simulink model "sm_car"  (R2022a)
settings: Solver=ode23t  StartTime=0.0  StopTime=200  MaxStep=0.4  RelTol=1e-3  AbsTol=1e-3  EnableMultiTasking=on
PreLoadFcn:
  | disp('Loading default data for 2-axle vehicle and 1-axle trailer.')
  | if verLessThan('matlab', '9.11')
  |     load Vehicle_139
  |     Vehicle = Vehicle_139;
  |     load Trailer_01
  |     Trailer = Trailer_01;
  | else
  |     load Vehicle_189
  |     Vehicle = Vehicle_189;
  |     load Trailer_07
  |     Trailer = Trailer_07;
  | end
  | 
  | disp('Turning off MFEval warnings...')
  | disp('Solver:CoeffChecks:Eyk -- OFF')
  | disp('Solver:Limits:Exceeded -- OFF')
  | disp('Solver:CoeffChecks:Et -- OFF')
  | disp('Solver:CoeffChecks:Exa -- OFF')
  | 
  | warning('off','Solver:CoeffChecks:Eyk')
  | warning('off','Solver:Limits:Exceeded')
  | warning('off','Solver:CoeffChecks:Et')
  | warning('off','Solver:CoeffChecks:Exa')
  | %warning('off','Solver:Radius:NegativeRho')
  | 
  | % Due to usability issue in Repeating Sequence block
  | warning('off','Simulink:Masking:Invalid');
  | 
  | % Eliminate unnecessary warnings in inactive variants
  | % Warnings generated only if you click through inactive variant
  | warning('off','MATLAB:nonExistentField');
  | warning('off','Simulink:Parameters:BlkParamUndefined');
PostLoadFcn:
  | disp('Disabling trailer by default.')
  | set_param([bdroot '/Vehicle'],'popup_trailer','Off')
  | warning('off','sm:sli:setup:compile:LocalSolverNotSupported')
  | sm_car_config_maneuver(bdroot,'WOT Braking');
  | sm_car_config_vehicle(bdroot);
  | sm_car_config_logging(bdroot);
InitFcn:
  | sm_car_config_camera;
  | Vehicle = sm_car_vehcfg_checkConfig(Vehicle);
  | sm_car_check_tire_model(bdroot);
  | addpath('C:\MasterThesis_CEVT\code\casadi-windows-matlabR2016a-v3.5.5')
  | addpath('C:\MasterThesis_CEVT\code')
  | addpath('C:\MasterThesis_CEVT\code\python scripts')
StartFcn:
  | tic;
StopFcn:
  | Elapsed_Sim_Time = toc;
  | % disp(['Elapsed Sim Time = ' num2str(Elapsed_Sim_Time)]);
  | % Run script that exports relevant simulation data to json
  | simToJson
undefined symbols (not defined in the file or in its folder): Control, Driver, Maneuver
libraries: sm_car_lib x22, simulink x17, sm_lib x3, Vehicle_Visualization x3, Driver_Long_Lat_Stanley x2, Maneuver_Get_Pose x2, Camera_Frame_Definitions x1, Control_FuelCell1Motor x1, slpidlib x1, Driver_Drive_Cycle x1, Driver_Gamepad_Xbox x1, Driver_Open_Loop x1
(part 2 of 3)

== system sm_car/Road/Input fWindTrailer ==
  Bus Creator1 : BusCreator  Inputs=3
  Demux : Demux  Outputs=3
  Scope : Scope
  Step : Step  Time=dWind  After=fWind  SampleTime=0
  Step1 : Step  Time=dWind+tWind  After=fWind  SampleTime=0
  Sum : Sum  Inputs=|+-
  fWind : Outport  VectorParamsAs1DForOutWhenUnconnected=off
  wires:
  Bus Creator1/1 -> fWind/1
  Demux/3 -> Bus Creator1/3  "fz"
  Demux/1 -> Bus Creator1/1  "fx"
  Demux/2 -> Bus Creator1/2  "fy"
  Sum/1 -> Scope/1, Demux/1  "fxyz"
  Step1/1 -> Sum/2
  Step/1 -> Sum/1

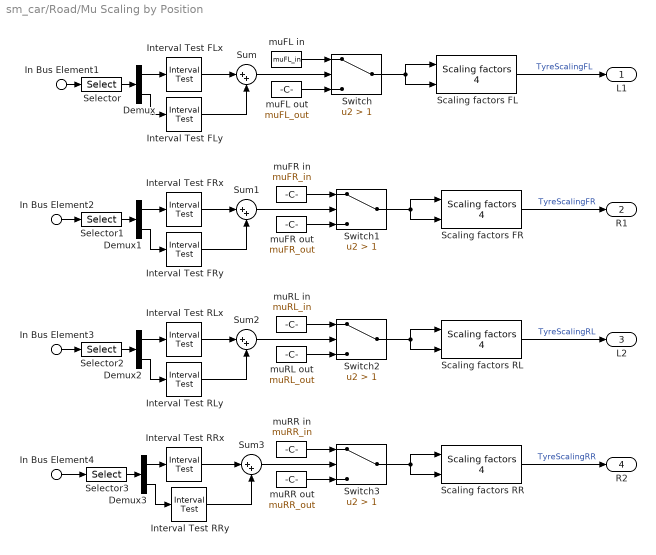
== system sm_car/Road/Mu Scaling by Position ==
  In Bus Element1 : Inport  PortName=Chassis  Element=WhlL1.xyz
  In Bus Element2 : Inport  PortName=Chassis  Element=WhlR1.xyz
  In Bus Element3 : Inport  PortName=Chassis  Element=WhlL2.xyz
  In Bus Element4 : Inport  PortName=Chassis  Element=WhlR2.xyz
  Demux{,1..3} (4 alike) : Demux  Outputs=2
  Interval Test FLx : simulink/Logic and Bit Operations/Interval Test  IntervalClosedRight=on  uplimit=intvX_FL_end  IntervalClosedLeft=on  lowlimit=intvX_FL_start  OutDataTypeStr=uint8
  Interval Test FLy : simulink/Logic and Bit Operations/Interval Test  IntervalClosedRight=on  uplimit=intvY_FL_end  IntervalClosedLeft=on  lowlimit=intvY_FL_start  OutDataTypeStr=uint8
  Interval Test FRx : simulink/Logic and Bit Operations/Interval Test  IntervalClosedRight=on  uplimit=intvX_FR_end  IntervalClosedLeft=on  lowlimit=intvX_FR_start  OutDataTypeStr=uint8
  Interval Test FRy : simulink/Logic and Bit Operations/Interval Test  IntervalClosedRight=on  uplimit=intvY_FR_end  IntervalClosedLeft=on  lowlimit=intvY_FR_start  OutDataTypeStr=uint8
  Interval Test RLx : simulink/Logic and Bit Operations/Interval Test  IntervalClosedRight=on  uplimit=intvX_RL_end  IntervalClosedLeft=on  lowlimit=intvX_RL_start  OutDataTypeStr=uint8
  Interval Test RLy : simulink/Logic and Bit Operations/Interval Test  IntervalClosedRight=on  uplimit=intvY_RL_end  IntervalClosedLeft=on  lowlimit=intvY_RL_start  OutDataTypeStr=uint8
  Interval Test RRx : simulink/Logic and Bit Operations/Interval Test  IntervalClosedRight=on  uplimit=intvX_RR_end  IntervalClosedLeft=on  lowlimit=intvX_RR_start  OutDataTypeStr=uint8
  Interval Test RRy : simulink/Logic and Bit Operations/Interval Test  IntervalClosedRight=on  uplimit=intvY_RR_end  IntervalClosedLeft=on  lowlimit=intvY_RR_start  OutDataTypeStr=uint8
  Scaling factors FL : sm_car_lib/Tires/Scaling factors 4  LKX=1  LKY=1  LKYC=1  LTR=1  LKZC=1
  Scaling factors FR : sm_car_lib/Tires/Scaling factors 4  LKX=1  LKY=1  LKYC=1  LTR=1  LKZC=1
  Scaling factors RL : sm_car_lib/Tires/Scaling factors 4  LKX=1  LKY=1  LKYC=1  LTR=1  LKZC=1
  Scaling factors RR : sm_car_lib/Tires/Scaling factors 4  LKX=1  LKY=1  LKYC=1  LTR=1  LKZC=1
  Selector{,1..3} (4 alike) : Selector  InputPortWidth=3  IndexOptions=Index vector (dialog)  Indices=[1 2]  OutputSizes=1
  Sum{,1..3} (4 alike) : Sum  Inputs=|++
  Switch : Switch  Criteria=u2 > Threshold  Threshold=1  ZeroCross=off  SaturateOnIntegerOverflow=off  InputSameDT=off
  Switch1 : Switch  Criteria=u2 > Threshold  Threshold=1  SaturateOnIntegerOverflow=off  InputSameDT=off
  Switch2 : Switch  Criteria=u2 > Threshold  Threshold=1  SaturateOnIntegerOverflow=off  InputSameDT=off
  Switch3 : Switch  Criteria=u2 > Threshold  Threshold=1  SaturateOnIntegerOverflow=off  InputSameDT=off
  muFL in : Constant  Value=muFL_in
  muFL out : Constant  Value=muFL_out
  muFR in : Constant  Value=muFR_in
  muFR out : Constant  Value=muFR_out
  muRL in : Constant  Value=muRL_in
  muRL out : Constant  Value=muRL_out
  muRR in : Constant  Value=muRR_in
  muRR out : Constant  Value=muRR_out
  L1 : Outport  VectorParamsAs1DForOutWhenUnconnected=off
  R1 : Outport  Port=2  VectorParamsAs1DForOutWhenUnconnected=off
  L2 : Outport  Port=3  VectorParamsAs1DForOutWhenUnconnected=off
  R2 : Outport  Port=4  VectorParamsAs1DForOutWhenUnconnected=off
  wires:
  Demux/1 -> Interval Test FLx/1
  Interval Test RRx/1 -> Sum3/1
  Demux3/2 -> Interval Test RRy/1
  Demux3/1 -> Interval Test RRx/1
  Sum3/1 -> Switch3/2
  Selector3/1 -> Demux3/1
  In Bus Element4/1 -> Selector3/1
  Interval Test RRy/1 -> Sum3/2
  Demux2/2 -> Interval Test RLy/1
  Selector2/1 -> Demux2/1
  Demux2/1 -> Interval Test RLx/1
  Interval Test RLy/1 -> Sum2/2
  Sum2/1 -> Switch2/2
  In Bus Element3/1 -> Selector2/1
  Interval Test RLx/1 -> Sum2/1
  Interval Test FRy/1 -> Sum1/2
  Selector1/1 -> Demux1/1
  Demux1/2 -> Interval Test FRy/1
  Sum1/1 -> Switch1/2
  Demux1/1 -> Interval Test FRx/1
  Interval Test FRx/1 -> Sum1/1
  Interval Test FLx/1 -> Sum/1
  Interval Test FLy/1 -> Sum/2
  Sum/1 -> Switch/2
  Demux/2 -> Interval Test FLy/1
  Selector/1 -> Demux/1
  muRR out/1 -> Switch3/3
  muRR in/1 -> Switch3/1
  Switch3/1 -> Scaling factors RR/2, Scaling factors RR/1
  Scaling factors RR/1 -> R2/1  "TyreScalingRR"
  Scaling factors RL/1 -> L2/1  "TyreScalingRL"
  Switch2/1 -> Scaling factors RL/1, Scaling factors RL/2
  muRL in/1 -> Switch2/1
  muRL out/1 -> Switch2/3
  muFR out/1 -> Switch1/3
  In Bus Element2/1 -> Selector1/1
  muFR in/1 -> Switch1/1
  Switch1/1 -> Scaling factors FR/2, Scaling factors FR/1
  Scaling factors FR/1 -> R1/1  "TyreScalingFR"
  Scaling factors FL/1 -> L1/1  "TyreScalingFL"
  Switch/1 -> Scaling factors FL/1, Scaling factors FL/2
  muFL out/1 -> Switch/3
  muFL in/1 -> Switch/1
  In Bus Element1/1 -> Selector/1

== system sm_car/Scopes/Subsystem ==
  In1 : Inport
  Bus Selector4 : BusSelector  OutputSignals=Chassis.Body.CG.vx,Chassis.Body.CG.vy,World.vx,World.vy,World.x,World.y
  Mux : Mux  Inputs=2
  Mux1 : Mux  Inputs=2
  Mux2 : Mux  Inputs=2
  Vel in xy plane : Fcn  Expr=sqrt(u(1)^2+u(2)^2)
  Vel in xy plane1 : Fcn  Expr=sqrt(u(1)^2+u(2)^2)
  Vel in xy plane2 : Fcn  Expr=sqrt(u(1)^2+u(2)^2)
  vBody : Outport  VectorParamsAs1DForOutWhenUnconnected=off
  vWorld : Outport  Port=2  VectorParamsAs1DForOutWhenUnconnected=off
  xWorld : Outport  Port=3  VectorParamsAs1DForOutWhenUnconnected=off
  wires:
  Bus Selector4/3 -> Mux1/1  "<vx>"
  Bus Selector4/4 -> Mux1/2  "<vy>"
  Bus Selector4/1 -> Mux/1  "<vx>"
  Vel in xy plane1/1 -> vWorld/1  "speed"
  In1/1 -> Bus Selector4/1
  Mux1/1 -> Vel in xy plane1/1
  Mux/1 -> Vel in xy plane/1
  Vel in xy plane/1 -> vBody/1  "speed"
  Bus Selector4/2 -> Mux/2  "<vy>"
  Mux2/1 -> Vel in xy plane2/1
  Bus Selector4/6 -> Mux2/2  "<y>"
  Bus Selector4/5 -> Mux2/1  "<x>"
  Vel in xy plane2/1 -> xWorld/1  "speed"

== system sm_car/Vehicle/Vehicle Constraint ==
  No Constraint : Subsystem  VariantControl=NoConstraint
  No Yaw : Subsystem  VariantControl=NoYaw
  F : PMIOPort  Side=Right
  B : PMIOPort  Port=2  Side=Left

== system sm_car/Visualization/Dashboard ==
  VehBus : Inport
  DrvBus : Inport  Port=2
  Accelerator Pedal : LinearGaugeBlock  LabelPosition=Hide  ScaleMax=1
  Brake Pedal : LinearGaugeBlock  ScaleMax=1
  Bus Selector : BusSelector  OutputSignals=Chassis.Body.CG.vx
  Bus Selector2 : BusSelector  OutputSignals=aSteerWheel,rAccelPedal,rBrakePedal
  Gain : Gain  Gain=180/pi
  Gain1 : Gain  Gain=3.6
  Speed (kph) : CustomWebBlock  LabelPosition=Hide  ShowInitialText=on  Configuration="{\"components\":[{\"name\":\"CircularScaleComponent\",\"settings\":{\"bounds\":{\"max\":150,\"min\":0,\"tickInterval\":\"auto\"},\"direction\":\"cw\",\"flipLimits\":0,\"innerRadius\":0.46396628518311167,\"internalTickHeightScaleFactor\":1,\"labelColor\":[250,245,200],\"labelFont\":{\"font\":\"Arial\",\"fontSize\":12},\"labelRadius\":0.36,\"labelTransparency\":1,\"minorTickHeightScaleFactor\":0.2,\"needleImage\":{\"size\":[1890,567],\"src\":\"data:image\\/svg+xml;base64,PD94bWwgdmVyc2lvbj0iMS4wIiBlbmNvZGluZz0iVVRGLTgiIHN0YW5kYWxvbmU9Im5vIj8+CjxzdmcKICAgeG1sbnM6ZGM9Imh0dHA6Ly9wdXJsLm9yZy9kYy9lbGVtZW50cy8xLjEvIgogICB4bWxuczpjYz0iaHR0cDovL2NyZWF0aXZlY29tbW9ucy5vcmcvbnMjIgogICB4bWxuczpyZGY9Imh0dHA6Ly93d3cudzMub3JnLzE5OTkvMDIvMjItcmRmLXN5bnRheC1ucyMiCiAgIHhtbG5zOnN2Zz0iaHR0cDovL3d3dy53My5vcmcvMjAwMC9zdmciCiAgIHhtbG5zPSJodHRwOi8vd3d3LnczLm9yZy8yMDAwL3N2ZyIKICAgeG1sbnM6 ...(+4096 chars)\"},\"needleOffset\":[0.14,0],\"needleOrientation\":-45,\"needleRotation\":180,\"needleSize\":{\"height\":0.13,\"width\":0.41},\"outerRadius\":0.6228849068763098,\"position\":[0,0,1,1],\"scaleAngle\":299.999999999988,\"scaleAngleOffset\":119.46147497096791,\"scaleColors\":[],\"scaleColorsSize\":0.2,\"scalePosition\":[0,0,1,1],\"showLabels\":1,\"showMinorTicks\":1,\"showSpanLine\":1,\"showTicks\":1,\"tickColor\":[250,245,200],\"tickTransparency\":1,\"valueBarColor\":[23,89,176],\"valueBarPosition\":[0,0,1,1],\"valueBarSize\":0.2,\"valueBarTransparency\":1}},{\"name\":\"BackgroundImageComponent\",\"settings\":{\"image\":{\"size\":[500,500],\"src\":\"data:image\\/svg+xml;base64,PD94bWwgdmVyc2lvbj0iMS4wIiBlbmNvZGluZz0iVVRGLTgiIHN0YW5kYWxvbmU9Im5vIj8+CjwhLS0gR2VuZXJhdG9yOiBBZG9iZSBJbGx1c3RyYXRvciAxOS4yLjEsIFNWRyBFeHBvcnQgUGx1Zy1JbiAuIFNWRyBWZXJzaW9uOiA2LjAwIEJ1aWxkIDApICAtLT4KCjxzdmcKICAgeG1sbnM6ZGM9Imh0dHA6Ly9wdXJsLm9yZy9kYy9lbGVtZW50cy8xLjEvIgogICB4bWxuczpjYz0iaHR0cDovL2NyZWF0aXZlY29tbW9ucy5vcmcvbnMjIgogICB4bWxuczpyZGY9Imh0dHA6Ly93d3cudzMub3JnLzE5OTkvMDIvMjItcmRmLXN5bnRh ...(+9660 chars)\",\"srcOrientation\":\"horizontal\"},\"position\":[0,0,1,1],\"scaleMode\":\"0\"}},{\"name\":\"ForegroundImageComponent\",\"settings\":{\"image\":{\"size\":[0,0],\"src\":\"default\",\"srcOrientation\":[]},\"isForeground\":1,\"position\":[0,0,1,1],\"scaleMode\":\"0\"}}],\"settings\":{\"BindingType\":\"signal\",\"backgroundOffset\":0.14,\"backgroundOpacity\":1,\"fixedAspectRatio\":\"on\",\"orientation\":\"horizontal\",\"showBackgroundColor\":0},\"type\":\"CircularGauge\"}"
  Steering Wheel Angle : SemiCircularGaugeBlock  LabelPosition=Hide  ScaleMin=-80  ScaleMax=80  TickInterval=20
  Terminator{,1..3} (4 alike) : Terminator
  wires:
  VehBus/1 -> Bus Selector/1
  DrvBus/1 -> Bus Selector2/1
  Bus Selector/1 -> Gain1/1  "<vx>"
  Gain/1 -> Terminator1/1  "aSteerWheel deg"
  Bus Selector2/3 -> Terminator3/1  "<rBrakePedal>"
  Bus Selector2/1 -> Gain/1  "<aSteerWheel>"
  Bus Selector2/2 -> Terminator2/1  "<rAccelPedal>"
  Gain1/1 -> Terminator/1  "Speed (kph)"

== system sm_car/Visualization/Unreal ==
  "xyz " : Inport
  "rpy " : Inport  Port=2
  "ws " : Inport  Port=3
  "aCamber " : Inport  Port=4
  "aSteerWheel " : Inport  Port=5
  Animation Off : Subsystem  VariantControl=Off
  Animation On : Subsystem  VariantControl=On

== system sm_car/Visualization/XY Plot ==
  "VehBus " : Inport
  "DrvBus " : Inport  Port=2
  XY Plot Off : Subsystem  VariantControl=Off
  XY Plot On : Vehicle_Visualization/XY Plot  SystemSampleTime=-1  VariantControl=On  VariantActivationTime=update diagram  Latency=0  AutoFrameSizeCalculation=off

== system sm_car/Controller/Battery 2 Motor/Accel Torque Request ==
  note: Convert Accelerator Pedal Position to Torque Command
      | using Motor Torque Speed Curve
  MotSpdA1 : Inport
  MotSpdA2 : Inport  Port=2
  AccelPdl : Inport  Port=3
  MaxMotTrqVsSpdA1 : Lookup_n-D  NumberOfTableDimensions=1  BreakpointsForDimension1=Control.MotorA1.TorqueSpd.w.Value %Mot.w_eff_bp_EV_rear  Table=Control.MotorA1.TorqueSpd.trq.Value % Mot.T_t_EV_rear  ExtrapMethod=Clip  UseLastTableValue=on  InternalRulePriority=Speed  OutDataTypeStr=Inherit: Inherit from 'Table data'  RndMeth=Simplest
  MaxMotTrqVsSpdA2 : Lookup_n-D  NumberOfTableDimensions=1  BreakpointsForDimension1=Control.MotorA2.TorqueSpd.w.Value  Table=Control.MotorA2.TorqueSpd.trq.Value  ExtrapMethod=Clip  UseLastTableValue=on  InternalRulePriority=Speed  OutDataTypeStr=Inherit: Inherit from 'Table data'  RndMeth=Simplest
  Mux : Mux  Inputs=2
  Product1 : Product
  Product2 : Product
  rads_to_rpm : Gain  Gain=30/pi
  rads_to_rpm1 : Gain  Gain=30/pi
  TrqCmd : Outport  VectorParamsAs1DForOutWhenUnconnected=off
  wires:
  rads_to_rpm/1 -> MaxMotTrqVsSpdA1/1
  MotSpdA1/1 -> rads_to_rpm/1
  AccelPdl/1 -> Product1/1, Product2/1
  MaxMotTrqVsSpdA1/1 -> Product1/2
  Product1/1 -> Mux/1
  MotSpdA2/1 -> rads_to_rpm1/1
  rads_to_rpm1/1 -> MaxMotTrqVsSpdA2/1
  MaxMotTrqVsSpdA2/1 -> Product2/2
  Product2/1 -> Mux/2
  Mux/1 -> TrqCmd/1

== system sm_car/Controller/Battery 2 Motor/Accel//Decel ==
  TrqCmdDec : Inport
  TrqCmdAcc : Inport  Port=2
  AccelPdl : Inport  Port=3
  Accel Decel Switch : Switch  Criteria=u2 > Threshold  SaturateOnIntegerOverflow=off  InputSameDT=off
  Compare To Constant : simulink/Logic and Bit Operations/Compare To Constant  relop=>  const=1e-2  OutDataTypeStr=boolean  ZeroCross=off
  Demux : Demux  Outputs=2
  MotTrqA1 : Outport  VectorParamsAs1DForOutWhenUnconnected=off
  MotTrqA2 : Outport  Port=2  VectorParamsAs1DForOutWhenUnconnected=off
  wires:
  TrqCmdDec/1 -> Accel Decel Switch/3
  Accel Decel Switch/1 -> Demux/1
  TrqCmdAcc/1 -> Accel Decel Switch/1
  AccelPdl/1 -> Compare To Constant/1
  Compare To Constant/1 -> Accel Decel Switch/2
  Demux/1 -> MotTrqA1/1
  Demux/2 -> MotTrqA2/1

== system sm_car/Controller/Battery 2 Motor/Battery Management System ==
  note: Behaviorial BMS System. Limits battery charge / discharge power based on SOC.
      |
      | Charge/Discharge Limits and curves can be adjusted if using a larger battery pack
      | or motor power is changed.
  SOC : Inport
  ChrgLmt : Lookup_n-D  NumberOfTableDimensions=1  BreakpointsForDimension1=Control.Battery.SOC_bpt  Table=Control.Battery.ChrgLmt_bpt  ExtrapMethod=Clip  UseLastTableValue=on  InternalRulePriority=Speed  RndMeth=Simplest
  DischrgLmt : Lookup_n-D  NumberOfTableDimensions=1  BreakpointsForDimension1=Control.Battery.SOC_bpt  Table=Control.Battery.DischrgLmt_bpt  ExtrapMethod=Clip  UseLastTableValue=on  InternalRulePriority=Speed  RndMeth=Simplest
  MaxChrg : Constant  Value=Control.Battery.BattChrgMax
  MaxDischrg : Constant  Value=Control.Battery.BattDischrgMax
  Product : Product
  Product1 : Product
  PwrLimtDis : Outport  VectorParamsAs1DForOutWhenUnconnected=off
  PwrLimitChg : Outport  Port=2  VectorParamsAs1DForOutWhenUnconnected=off
  wires:
  DischrgLmt/1 -> Product/1
  ChrgLmt/1 -> Product1/1
  Product1/1 -> PwrLimitChg/1
  Product/1 -> PwrLimtDis/1
  MaxDischrg/1 -> Product/2
  MaxChrg/1 -> Product1/2
  SOC/1 -> ChrgLmt/1, DischrgLmt/1

== system sm_car/Controller/Battery 2 Motor/Brake Pressure Request ==
  note: Converts Brake Pedal Position to Deceleration Request
  DecelPdl : Inport
  Park : Inport  Port=2
  Constant1 : Constant
  Switch : Switch  Criteria=u2 > Threshold  ZeroCross=off  SaturateOnIntegerOverflow=off  InputSameDT=off
  BrkDecelReq : Outport  VectorParamsAs1DForOutWhenUnconnected=off
  wires:
  Park/1 -> Switch/2
  Switch/1 -> BrkDecelReq/1
  Constant1/1 -> Switch/1
  DecelPdl/1 -> Switch/3

== system sm_car/Controller/Battery 2 Motor/Per wheel ==
  pBrake : Inport
  Bus Creator4 : BusCreator  Inputs=4
  Gain1 : Gain  Gain=0.6
  Gain2 : Gain  Gain=0.6
  Gain3 : Gain  Gain=0.4
  Gain4 : Gain  Gain=0.4
  Gain5 : Gain  Gain=0.5
  Transfer Fcn : TransferFcn  Denominator=[0.01 1]
  p : Outport  VectorParamsAs1DForOutWhenUnconnected=off
  wires:
  Gain4/1 -> Bus Creator4/4  "pBrakeR2"
  Gain3/1 -> Bus Creator4/3  "pBrakeL2"
  Gain1/1 -> Bus Creator4/2  "pBrakeR1"
  Bus Creator4/1 -> p/1
  pBrake/1 -> Transfer Fcn/1
  Gain2/1 -> Bus Creator4/1  "pBrakeL1"
  Gain5/1 -> Gain2/1, Gain1/1, Gain3/1, Gain4/1  "pBrakeL1"
  Transfer Fcn/1 -> Gain5/1

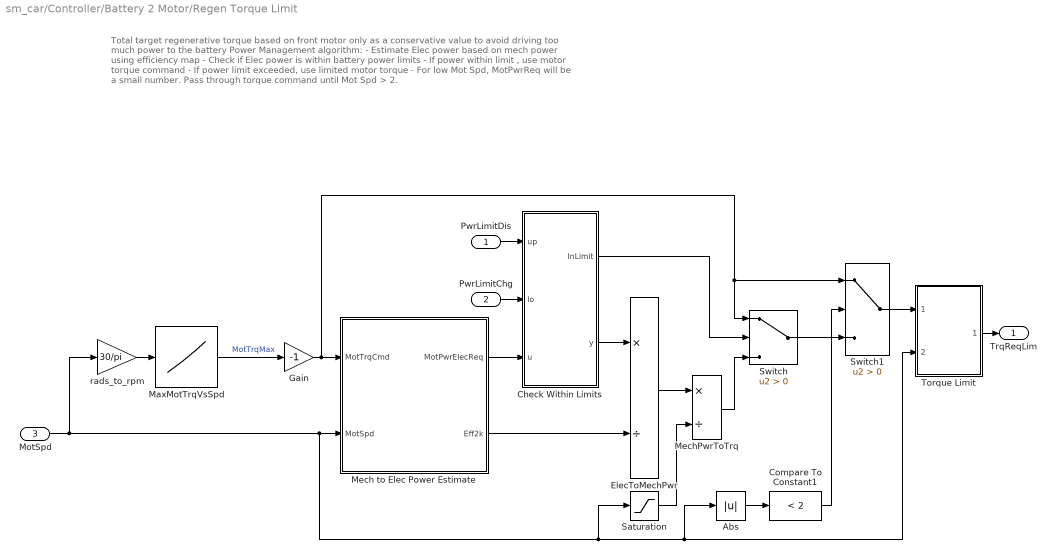
== system sm_car/Controller/Battery 2 Motor/Regen Torque Limit ==
  note: Total target regenerative torque based on front motor only as a conservative value to avoid driving too much power to the battery
      |
      | Power Management algorithm:
      | - Estimate Elec power based on mech power using efficiency map
      | - Check if Elec power is within battery power limits
      | - If power within limit , use motor torque command
      | - If power limit exceeded, use limited motor torque
      | - For low Mot Spd, MotPwrReq will be a small number.  Pass through torque command until Mot Spd > 2.
  PwrLimitDis : Inport
  "PwrLimitChg " : Inport  Port=2
  MotSpd : Inport  Port=3
  Abs : Abs  ZeroCross=off  SaturateOnIntegerOverflow=off
  Check Within Limits : Subsystem
  Compare To Constant1 : simulink/Logic and Bit Operations/Compare To Constant  relop=<  const=2  OutDataTypeStr=boolean  ZeroCross=off
  ElecToMechPwr : Product  Inputs=*/
  Gain : Gain  Gain=-1
  MaxMotTrqVsSpd : Lookup_n-D  NumberOfTableDimensions=1  BreakpointsForDimension1=Control.MotorA1.TorqueSpd.w.Value  Table=Control.MotorA1.TorqueSpd.trq.Value  ExtrapMethod=Clip  UseLastTableValue=on  InternalRulePriority=Speed  OutDataTypeStr=Inherit: Inherit from 'Table data'  RndMeth=Simplest
  Mech to Elec Power Estimate : Subsystem
  MechPwrToTrq : Product  Inputs=*/
  Saturation : Saturate  UpperLimit=inf  LowerLimit=2
  Switch : Switch  Criteria=u2 > Threshold  ZeroCross=off  SaturateOnIntegerOverflow=off  InputSameDT=off
  Switch1 : Switch  Criteria=u2 > Threshold  ZeroCross=off  SaturateOnIntegerOverflow=off  InputSameDT=off
  Torque Limit : Subsystem
  rads_to_rpm : Gain  Gain=30/pi
  "TrqReqLim " : Outport  VectorParamsAs1DForOutWhenUnconnected=off
  wires:
  Switch1/1 -> Torque Limit/1(MotTrq)
  Torque Limit/1(MotReqCmd) -> "TrqReqLim "/1
  Mech to Elec Power Estimate/2(Eff2k) -> ElecToMechPwr/2
  PwrLimitDis/1 -> Check Within Limits/1(up)
  "PwrLimitChg "/1 -> Check Within Limits/2(lo)
  Gain/1 -> Mech to Elec Power Estimate/1(MotTrqCmd), Switch/1, Switch1/1
  Check Within Limits/1(InLimit) -> Switch/2
  Check Within Limits/2(y) -> ElecToMechPwr/1
  Mech to Elec Power Estimate/1(MotPwrElecReq) -> Check Within Limits/3(u)
  Switch/1 -> Switch1/3
  Abs/1 -> Compare To Constant1/1
  Compare To Constant1/1 -> Switch1/2
  Saturation/1 -> MechPwrToTrq/2
  MechPwrToTrq/1 -> Switch/3
  ElecToMechPwr/1 -> MechPwrToTrq/1
  rads_to_rpm/1 -> MaxMotTrqVsSpd/1
  MaxMotTrqVsSpd/1 -> Gain/1  "MotTrqMax"
  MotSpd/1 -> Torque Limit/2(MotSpd), Abs/1, Saturation/1, Mech to Elec Power Estimate/2(MotSpd), rads_to_rpm/1

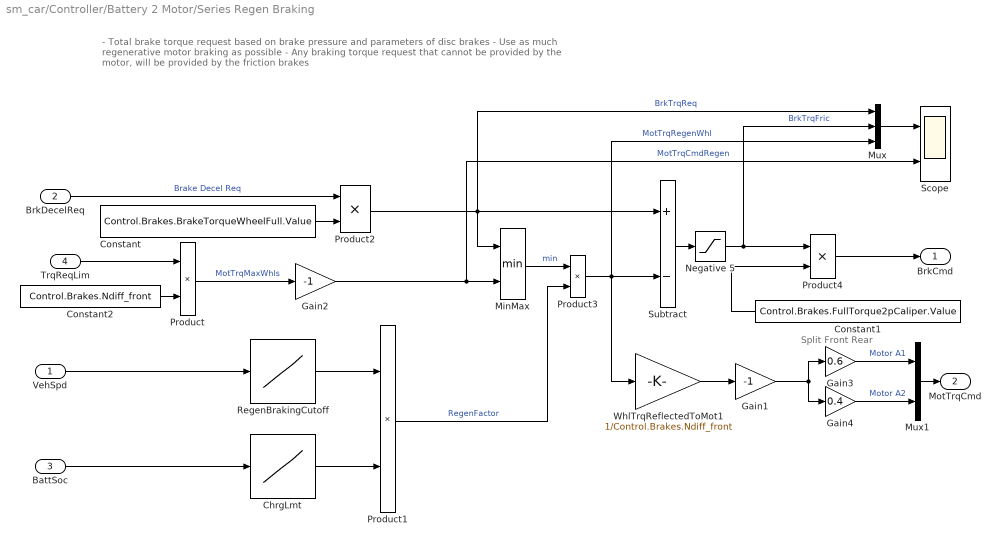
== system sm_car/Controller/Battery 2 Motor/Series Regen Braking ==
  note: Split Front Rear
  note: - Total brake torque request based on brake pressure and parameters of disc brakes
      | - Use as much regenerative motor braking as possible
      | - Any braking torque request that cannot be provided by the motor, will be provided by the friction brakes
  VehSpd : Inport
  BrkDecelReq : Inport  Port=2
  BattSoc : Inport  Port=3
  TrqReqLim : Inport  Port=4
  ChrgLmt : Lookup_n-D  NumberOfTableDimensions=1  BreakpointsForDimension1=Control.Battery.SOC_bpt  Table=Control.Battery.ChrgLmt_bpt  ExtrapMethod=Clip  UseLastTableValue=on  InternalRulePriority=Speed  RndMeth=Simplest
  Constant : Constant  Value=Control.Brakes.BrakeTorqueWheelFull.Value
  Constant1 : Constant  Value=Control.Brakes.FullTorque2pCaliper.Value
  Constant2 : Constant  Value=Control.Brakes.Ndiff_front
  Gain1 : Gain  Gain=-1
  Gain2 : Gain  Gain=-1
  Gain3 : Gain  Gain=0.6
  Gain4 : Gain  Gain=0.4
  MinMax : MinMax  Inputs=2
  Mux : Mux  Inputs=3
  Mux1 : Mux  Inputs=2
  Negative 5 : Saturate  UpperLimit=inf  LowerLimit=0  ZeroCross=off
  Product{,1..3} (4 alike) : Product
  Product4 : Product  Inputs=**
  RegenBrakingCutoff : Lookup_n-D  NumberOfTableDimensions=1  BreakpointsForDimension1=Control.Power.RegenBrkSpd_bpt  Table=Control.Power.RegenBrkCutOff  ExtrapMethod=Clip  UseLastTableValue=on  InternalRulePriority=Speed  RndMeth=Simplest
  Scope : Scope  NumInputPorts=2
  Subtract : Sum  Inputs=+-
  WhlTrqReflectedToMot1 : Gain  Gain=1/Control.Brakes.Ndiff_front
  " BrkCmd" : Outport  VectorParamsAs1DForOutWhenUnconnected=off
  " MotTrqCmd" : Outport  Port=2  VectorParamsAs1DForOutWhenUnconnected=off
  wires:
  Product4/1 -> " BrkCmd"/1
  Negative 5/1 -> Product4/1, Mux/2  "BrkTrqFric"
  BattSoc/1 -> ChrgLmt/1
  Subtract/1 -> Negative 5/1
  Product1/1 -> Product3/2  "RegenFactor"
  RegenBrakingCutoff/1 -> Product1/1
  VehSpd/1 -> RegenBrakingCutoff/1
  ChrgLmt/1 -> Product1/2
  MinMax/1 -> Product3/1  "min"
  Product2/1 -> MinMax/1, Subtract/1, Mux/1  "BrkTrqReq"
  BrkDecelReq/1 -> Product2/1  "Brake Decel Req"
  Constant/1 -> Product2/2
  Constant1/1 -> Product4/2
  Product3/1 -> WhlTrqReflectedToMot1/1, Subtract/2, Mux/3  "MotTrqRegenWhl"
  Mux/1 -> Scope/1
  TrqReqLim/1 -> Product/1
  WhlTrqReflectedToMot1/1 -> Gain1/1
  Gain1/1 -> Gain3/1, Gain4/1
  Gain2/1 -> MinMax/2, Scope/2  "MotTrqCmdRegen"
  Product/1 -> Gain2/1  "MotTrqMaxWhls"
  Gain3/1 -> Mux1/1  "Motor A1"
  Gain4/1 -> Mux1/2  "Motor A2"
  Mux1/1 -> " MotTrqCmd"/1
  Constant2/1 -> Product/2

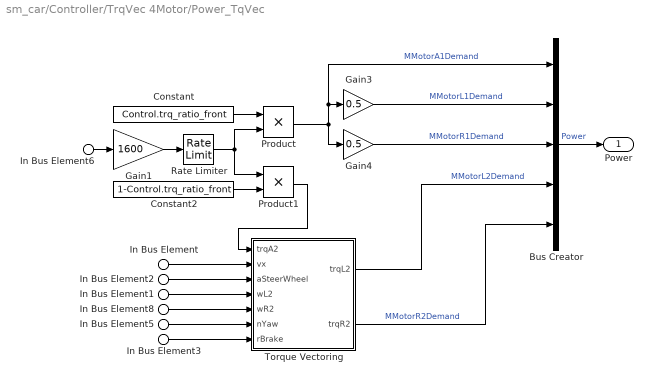
== system sm_car/Controller/TrqVec 4Motor/Power_TqVec ==
  In Bus Element6 : Inport  PortName=DrvBus  Element=rAccelPedal
  In Bus Element2 : Inport  PortName=DrvBus  Element=aSteerWheel
  In Bus Element3 : Inport  PortName=DrvBus  Element=rBrakePedal
  In Bus Element : Inport  Port=2  PortName=VehBus  Element=Chassis.Body.CG.vx
  In Bus Element1 : Inport  Port=2  PortName=VehBus  Element=Power.MotorL2.w
  In Bus Element8 : Inport  Port=2  PortName=VehBus  Element=Power.MotorR2.w
  In Bus Element5 : Inport  Port=2  PortName=VehBus  Element=World.nYaw
  Bus Creator : BusCreator  Inputs=5
  Constant : Constant  Value=Control.trq_ratio_front
  Constant2 : Constant  Value=1-Control.trq_ratio_front
  Gain1 : Gain  Gain=1600
  Gain3 : Gain  Gain=0.5
  Gain4 : Gain  Gain=0.5
  Product : Product
  Product1 : Product
  Rate Limiter : RateLimiter  RisingSlewLimit=300  FallingSlewLimit=-5000  SampleTimeMode=inherited
  Torque Vectoring : Subsystem  mask(Torque Vectoring, Rear Wheels){vx_enable=2.5, aSteerWheel_enable=4*pi/180, aStr_to_aWhl=0.33, max_torque_delta=200, P=4000, I=100}
      mask prompts: vx_enable "Speed to enable (m/s)"; aSteerWheel_enable "Steering wheel angle to enable (rad)"; aStr_to_aWhl "Steering Ratio (Wheel/Steering Wheel)"; max_torque_delta "Max Torque Split (N*m)"; P "Simulink:masks:ProportionalP_MP"; I "Simulink:masks:IntegralI_MP"
      mask help: Basic torque vectoring algorithm which applies opposing offsets to the commanded torque of the rear wheels based on the error between the vehicle slip angle and the angle of the steered wheels.
      mask TypeOptions vx_enable: Enable/Enable vx/const
      mask TypeOptions aSteerWheel_enable: Enable/Enable aSteerWheel/const
      mask TypeOptions aStr_to_aWhl:
      | Vehicle Slip Angle Error/Steering Wheel
      | to Driving Wheel/Gain
      mask TypeOptions max_torque_delta: Max Delta Torque/Value
      mask TypeOptions P: PID Controller/P
      mask TypeOptions I: PID Controller/I
      mask DialogControl P Prompt: Proportional (P):
      mask DialogControl I Prompt: Integral (I):
  Power : Outport  VectorParamsAs1DForOutWhenUnconnected=off
  wires:
  Gain1/1 -> Rate Limiter/1
  In Bus Element6/1 -> Gain1/1
  Rate Limiter/1 -> Product1/1, Product/2
  Constant/1 -> Product/1
  Constant2/1 -> Product1/2
  Product/1 -> Bus Creator/1, Gain3/1, Gain4/1  "MMotorA1Demand"
  Gain3/1 -> Bus Creator/2  "MMotorL1Demand"
  Gain4/1 -> Bus Creator/3  "MMotorR1Demand"
  Bus Creator/1 -> Power/1  "Power"
  Product1/1 -> Torque Vectoring/1(trqA2)
  In Bus Element/1 -> Torque Vectoring/2(vx)
  In Bus Element2/1 -> Torque Vectoring/3(aSteerWheel)
  In Bus Element1/1 -> Torque Vectoring/4(wL2)
  In Bus Element8/1 -> Torque Vectoring/5(wR2)
  In Bus Element5/1 -> Torque Vectoring/6(nYaw)
  In Bus Element3/1 -> Torque Vectoring/7(rBrake)
  Torque Vectoring/1(trqL2) -> Bus Creator/4  "MMotorL2Demand"
  Torque Vectoring/2(trqR2) -> Bus Creator/5  "MMotorR2Demand"

== system sm_car/Driver/Closed Loop/Scopes ==
  <vx> : Inport
  Ref : Inport  Port=2
  CurPose : Inport  Port=3
  DrvBus : Inport  Port=4
  Bus Selector1 : BusSelector  OutputSignals=aSteerWheel,rAccelPedal,rBrakePedal
  Compare vx to Target : Scope  NumInputPorts=2
  RefPose : Scope
  Scope1 : Scope  NumInputPorts=3
  wires:
  Ref/1 -> Compare vx to Target/2
  CurPose/1 -> RefPose/1
  Bus Selector1/3 -> Scope1/3  "<rBrakePedal>"
  <vx>/1 -> Compare vx to Target/1
  Bus Selector1/2 -> Scope1/2  "<rAccelPedal>"
  Bus Selector1/1 -> Scope1/1  "<aSteerWheel>"
  DrvBus/1 -> Bus Selector1/1

== system sm_car/Driver/Interactive/Pace Car ==
  "VehBus " : Inport
  None : Subsystem  VariantControl=None
  Show : Subsystem  VariantControl=Show

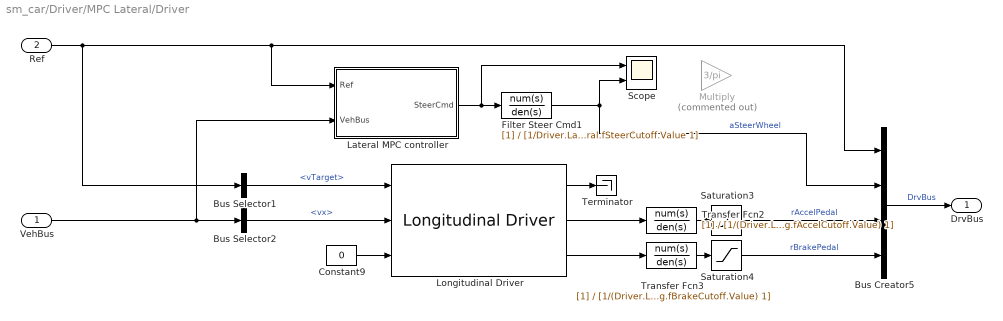
== system sm_car/Driver/MPC Lateral/Driver ==
  VehBus : Inport
  Ref : Inport  Port=2
  Bus Creator5 : BusCreator  Inputs=4
  Bus Selector1 : BusSelector  OutputSignals=vTarget
  Bus Selector2 : BusSelector  OutputSignals=Chassis.Body.CG.vx
  Constant9 : Constant  Value=0
  Filter Steer Cmd1 : TransferFcn  Denominator=[1/Driver.Lateral.fSteerCutoff.Value 1]
  Lateral MPC controller : Subsystem
  Longitudinal Driver : Driver_Long_Lat_Stanley/Long Lat Stanley/Longitudinal Driver  extAccelOvr=off  extDecelOvr=off  extAccelHld=off  extDecelHld=off  extAccelZero=off  extDecelZero=off  cntrlType=Predictive  shftType=None  velUnits=m/s  gearOut=off  Kp=15  Ki=1  Kff=.05  Kg=.01  VehVelVec=[0 100]  KffVec=[.1 .1]  KpVec=[10 10]  KiVec=[5 5]  KgVec=[0 0]  m=Driver.Long.mVehicle.Value  Kpt=Driver.Long.FTractive.Value  tau=Driver.Long.tDriver.Value  L=Driver.Long.xPreview.Value  aR=Driver.Long.NDragRoll.Value  bR=Driver.Long.NDragRollDriveline.Value  cR=Driver.Long.NDragAero.Value  g=Driver.Long.gGravity.Value  vnom=100  Kaw=.1  tauerr=.03  tauPt=2  GearInit=0  tShift=.1  pdlVec=[0.1 0.4 0.5 0.9]  upShftTbl=[-1 12.9375 26.4375 39.9375 51.18749999999999 62.4375 72.84375 83.25;-1 16.3125 29.8125 43.3125 54.5624 65.8125 76.78125 87.75;-1 19.6875 33.1875 46.68749999999999 57.9375 69.1875 80.71875 92.25;-1 33 52.5 77.25 100.5 138.75 161.875 185]  dwnShftTbl=[1 9.5625 23.0625 36.5625 47.8125 59.0625 68.90625 78.75;1 12.9375 26.4375 39.9375 51.18749999999999 62.4375 72.84375 83.25;1 16.3125 29.8125 43.3125 54.562499 65.8125 76.78125 87.75;1 19.6875 33.1875 46.68749999999999 57.9375 69.1875 80.71875 92.25]  tClutch=.5  tRev=.5  tPark=120  aMode=1  UpGearVec="[0  1  2  3  4  5  6  7]"  DownGearVec="[1  2  3  4  5  6  7  8]"
  Multiply : Gain  Commented=on  Gain=3/pi
  Saturation3 : Saturate  UpperLimit=1  LowerLimit=0  ZeroCross=off
  Saturation4 : Saturate  UpperLimit=1  LowerLimit=0  ZeroCross=off
  Scope : Scope  NumInputPorts=2
  Terminator : Terminator
  Transfer Fcn2 : TransferFcn  Denominator=[1/(Driver.Long.fAccelCutoff.Value) 1]
  Transfer Fcn3 : TransferFcn  Denominator=[1/(Driver.Long.fBrakeCutoff.Value) 1]
  DrvBus : Outport  VectorParamsAs1DForOutWhenUnconnected=off
  wires:
  Ref/1 -> Bus Selector1/1, Lateral MPC controller/1(Ref), Bus Creator5/1
  Bus Selector2/1 -> Longitudinal Driver/2  "<vx>"
  Bus Selector1/1 -> Longitudinal Driver/1  "<vTarget>"
  Bus Creator5/1 -> DrvBus/1  "DrvBus"
  VehBus/1 -> Lateral MPC controller/2(VehBus), Bus Selector2/1
  Filter Steer Cmd1/1 -> Scope/2, Bus Creator5/2  "aSteerWheel"
  Lateral MPC controller/1(SteerCmd) -> Scope/1, Filter Steer Cmd1/1
  Constant9/1 -> Longitudinal Driver/3
  Longitudinal Driver/2 -> Transfer Fcn2/1
  Saturation3/1 -> Bus Creator5/3  "rAccelPedal"
  Longitudinal Driver/3 -> Transfer Fcn3/1
  Saturation4/1 -> Bus Creator5/4  "rBrakePedal"
  Longitudinal Driver/1 -> Terminator/1
  Transfer Fcn3/1 -> Saturation4/1
  Transfer Fcn2/1 -> Saturation3/1

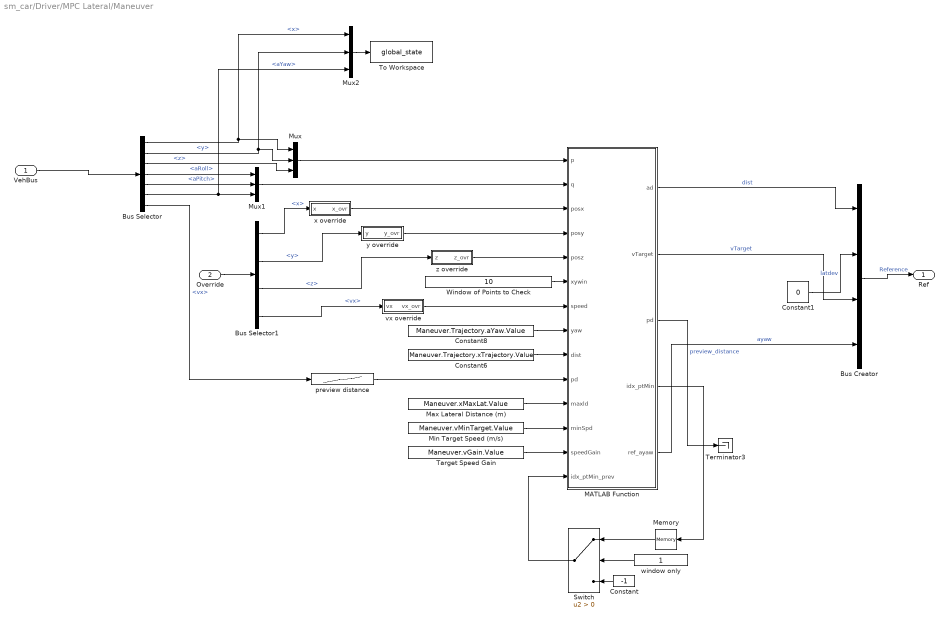
== system sm_car/Driver/MPC Lateral/Maneuver ==
  VehBus : Inport
  Override : Inport  Port=2
  Bus Creator : BusCreator  Inputs=4
  Bus Selector : BusSelector  OutputSignals=World.x,World.y,World.z,World.aRoll,World.aPitch,World.aYaw,Chassis.Body.CG.vx
  Bus Selector1 : BusSelector  OutputSignals=x,y,z,vx
  Constant : Constant  Value=-1
  Constant1 : Constant  Value=0
  Constant6 : Constant  Value=Maneuver.Trajectory.xTrajectory.Value
  Constant8 : Constant  Value=Maneuver.Trajectory.aYaw.Value
  MATLAB Function : MATLAB Function  SystemSampleTime=0.1
  Max Lateral Distance (m) : Constant  Value=Maneuver.xMaxLat.Value
  Memory : Memory  InitialCondition=-1
  Min Target Speed (m/s) : Constant  Value=Maneuver.vMinTarget.Value
  Mux : Mux  Inputs=3
  Mux1 : Mux  Inputs=3
  Mux2 : Mux  Inputs=3
  Switch : Switch  Criteria=u2 > Threshold  SaturateOnIntegerOverflow=off  InputSameDT=off
  Target Speed Gain : Constant  Value=Maneuver.vGain.Value
  Terminator3 : Terminator
  To Workspace : ToWorkspace  VariableName=global_state  SaveFormat=Structure With Time  SampleTime=0.1
  Window of Points to Check : Constant  Value=10
  preview distance : Lookup_n-D  NumberOfTableDimensions=1  BreakpointsForDimension1=Maneuver.xPreview.v.Value  Table=Maneuver.xPreview.x.Value  InternalRulePriority=Speed  RndMeth=Simplest
  vx override : Subsystem
  window only : Constant
  x override : Subsystem
  y override : Subsystem
  z override : Subsystem
  Ref : Outport  VectorParamsAs1DForOutWhenUnconnected=off
  wires:
  Mux1/1 -> MATLAB Function/2(q)
  Mux/1 -> MATLAB Function/1(p)
  Bus Selector1/1 -> x override/1(x)  "<x>"
  Bus Selector1/2 -> y override/1(y)  "<y>"
  Bus Selector1/3 -> z override/1(z)  "<z>"
  vx override/1(vx_ovr) -> MATLAB Function/7(speed)
  Bus Selector1/4 -> vx override/1(vx)  "<vx>"
  Override/1 -> Bus Selector1/1
  z override/1(z_ovr) -> MATLAB Function/5(posz)
  Memory/1 -> Switch/1
  window only/1 -> Switch/2
  Constant/1 -> Switch/3
  Switch/1 -> MATLAB Function/14(idx_ptMin_prev)
  MATLAB Function/4(idx_ptMin) -> Memory/1
  Window of Points to Check/1 -> MATLAB Function/6(xywin)
  MATLAB Function/2(vTarget) -> Bus Creator/3  "vTarget"
  Bus Creator/1 -> Ref/1  "Reference"
  MATLAB Function/1(ad) -> Bus Creator/1  "dist"
  VehBus/1 -> Bus Selector/1
  preview distance/1 -> MATLAB Function/10("pd ")
  x override/1(x_ovr) -> MATLAB Function/3(posx)
  Bus Selector/2 -> Mux2/2, Mux/2  "<y>"
  y override/1(y_ovr) -> MATLAB Function/4(posy)
  Bus Selector/3 -> Mux/3  "<z>"
  Constant6/1 -> MATLAB Function/9(dist)
  Bus Selector/5 -> Mux1/2  "<aPitch>"
  Bus Selector/7 -> preview distance/1  "<vx>"
  Constant8/1 -> MATLAB Function/8(yaw)
  Bus Selector/4 -> Mux1/1  "<aRoll>"
  Bus Selector/6 -> Mux2/3, Mux1/3  "<aYaw>"
  Bus Selector/1 -> Mux2/1, Mux/1  "<x>"
  Max Lateral Distance (m)/1 -> MATLAB Function/11(maxld)
  Target Speed Gain/1 -> MATLAB Function/13(speedGain)
  Min Target Speed (m/s)/1 -> MATLAB Function/12(minSpd)
  Mux2/1 -> To Workspace/1
  MATLAB Function/3(pd) -> Terminator3/1  "preview_distance"
  Constant1/1 -> Bus Creator/2  "latdev"
  MATLAB Function/5(ref_ayaw) -> Bus Creator/4  "ayaw"

== system sm_car/Driver/MPC Lateral/Scopes ==
  <vx> : Inport
  Ref : Inport  Port=2
  CurPose : Inport  Port=3
  DrvBus : Inport  Port=4
  Bus Selector1 : BusSelector  OutputSignals=aSteerWheel,rAccelPedal,rBrakePedal
  Compare vx to Target : Scope  NumInputPorts=2
  RefPose : Scope
  Scope1 : Scope  NumInputPorts=3
  wires:
  Ref/1 -> Compare vx to Target/2
  CurPose/1 -> RefPose/1
  Bus Selector1/3 -> Scope1/3  "<rBrakePedal>"
  <vx>/1 -> Compare vx to Target/1
  Bus Selector1/2 -> Scope1/2  "<rAccelPedal>"
  Bus Selector1/1 -> Scope1/1  "<aSteerWheel>"
  DrvBus/1 -> Bus Selector1/1

== system sm_car/Vehicle/Vehicle Constraint/No Constraint ==
  F : PMIOPort  Side=Right
  B : PMIOPort  Port=2  Side=Left
